simulink model "terrainfollow_debug"  (R2018a)
settings: Solver=VariableStepAuto  StartTime=0.0  StopTime=100  FixedStep=0.00001  RelTol=1e-3
values from neighbouring files (symbols this model uses):
  A = [0 0 0.00013165266625 3.15369085605e-06 -1.52707114267e-20 299.999999993 0 -32.1699999992 -6.02299064272e-14 0 0 0 ... (25 elements, 5x5)]    [redu_ss_terrainfollow.mat]    (also in reducefun_terrainfollow.m = A_lon_ac)
  B = [0  0; 0  0; 0.00154396044469  -0.00453382204302; -9.49308816068e-07  -0.00111635553349; 0  -0.0570163434913]    [redu_ss_terrainfollow.mat]    (also in reducefun_terrainfollow.m = B_lon_ac)
  C = [1 0 0 0 0 0 1 0 0 0 0 0 ... (25 elements, 5x5)]    [redu_ss_terrainfollow.mat]    (also in reducefun_terrainfollow.m = C_lon_ac)
  D = [0  0; 0  0; 0  0; 0  0; 0  0]    [redu_ss_terrainfollow.mat]    (also in reducefun_terrainfollow.m = D_lon_ac)
  ele_lowlim = -25    - de0    [terrainfollow_run.m]    (also in terrainfollow_sim_bigcanyon.m)
  ele_uplim = 25     - de0    [terrainfollow_run.m]    (also in terrainfollow_sim_bigcanyon.m)
  h0 = 1500    [terrainfollow_run.m]    (also in terrainfollow_sim_bigcanyon.m)
  K_f = lqr(A,B,Q_f,R_f)    [terrainfollow_run.m]    (also in terrainfollow_sim_bigcanyon.m)
  th_lowlim = 1000   - th0    [terrainfollow_run.m]    (also in terrainfollow_sim_bigcanyon.m)
  th_uplim = 19000  - th0    [terrainfollow_run.m]    (also in terrainfollow_sim_bigcanyon.m)
  v0 = ft2m*trim_state_lo(7)    [terrainfollow_run.m]    (also in terrainfollow_sim_bigcanyon.m)
libraries: aerolibconvert2 x4
settings Model: Creator=Lukas  LastModifiedBy=Lukas
settings CodeAppCC: StateflowObjectComments=on

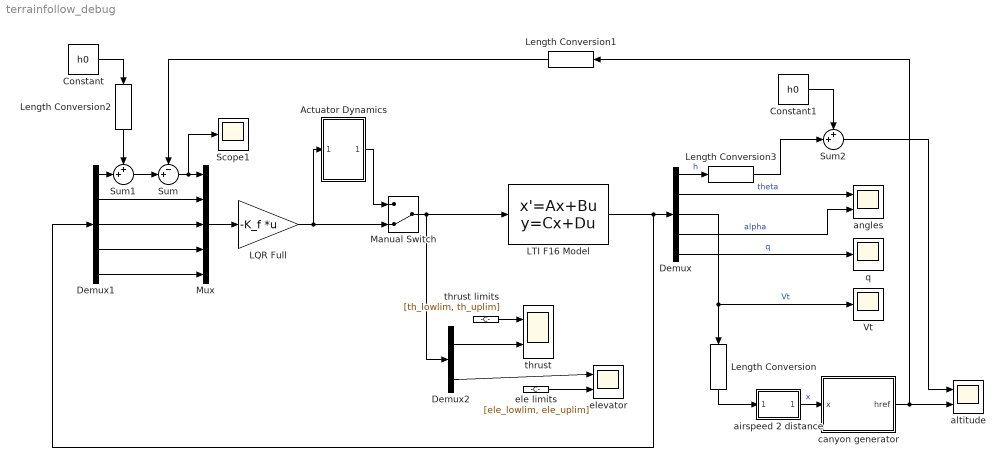
== system terrainfollow_debug ==
  Actuator Dynamics : Subsystem
  Constant : Constant  Value=h0
  Constant1 : Constant  Value=h0
  Demux : Demux  Outputs=5
  Demux1 : Demux  Outputs=5
  Demux2 : Demux  Outputs=2
  LQR Full : Gain  Gain=-K_f  Multiplication=Matrix(K*u)  SaturateOnIntegerOverflow=on  OutDataTypeStr=Inherit: Same as input  ParamDataTypeStr=Inherit: Same as input
  "LTI F16 Model " : StateSpace  A=A  B=B  C=C  D=D  InitialCondition=0
      mask Display: image('f16thumb.jpg');
  Length Conversion : aerolibconvert2/Length Conversion  IU=ft  OU=m
  Length Conversion1 : aerolibconvert2/Length Conversion  IU=m  OU=ft
  Length Conversion2 : aerolibconvert2/Length Conversion  IU=m  OU=ft
  Length Conversion3 : aerolibconvert2/Length Conversion  IU=ft  OU=m
  Manual Switch : ManualSwitch  CurrentSetting=0
  Mux : Mux  Inputs=5
  Scope1 : Scope
  Sum : Sum  Inputs=-+|
  Sum1 : Sum  Inputs=++|
  Sum2 : Sum  Inputs=++|
  Vt : Scope
  airspeed 2 distance : Subsystem
  altitude : Scope  NumInputPorts=2
  angles : Scope  NumInputPorts=2
  canyon generator : Subsystem
      mask Display: image(imread('canyon.jpg'))
  ele limits : Constant  Value=[ele_lowlim, ele_uplim]
  elevator : Scope  NumInputPorts=2
  q : Scope
  thrust : Scope  NumInputPorts=2
  thrust limits : Constant  Value=[th_lowlim, th_uplim]
  wires:
  "LTI F16 Model "/1 -> Demux1/1, Demux/1
  airspeed 2 distance/1(Out1) -> canyon generator/1(x)  "x"
  Demux/2 -> angles/1  "theta"
  Demux/5 -> q/1  "q"
  Demux/1 -> Length Conversion3/1  "h"
  Demux/3 -> Vt/1, Length Conversion/1  "Vt"
  Demux/4 -> angles/2  "alpha"
  Demux1/5 -> Mux/5
  Demux1/3 -> Mux/3
  Demux1/4 -> Mux/4
  Demux1/2 -> Mux/2
  Mux/1 -> LQR Full/1
  Demux1/1 -> Sum1/2
  Sum/1 -> Scope1/1, Mux/1
  canyon generator/1(href) -> Length Conversion1/1, altitude/2
  Sum1/1 -> Sum/2
  Constant/1 -> Length Conversion2/1
  Sum2/1 -> altitude/1
  Constant1/1 -> Sum2/1
  LQR Full/1 -> Manual Switch/2, Actuator Dynamics/1(In1)
  Actuator Dynamics/1(Out1) -> Manual Switch/1
  Manual Switch/1 -> "LTI F16 Model "/1, Demux2/1
  Length Conversion/1 -> airspeed 2 distance/1(In1)
  Length Conversion1/1 -> Sum/1
  Length Conversion2/1 -> Sum1/1
  Length Conversion3/1 -> Sum2/2
  Demux2/1 -> thrust/2
  Demux2/2 -> elevator/1
  thrust limits/1 -> thrust/1
  ele limits/1 -> elevator/2

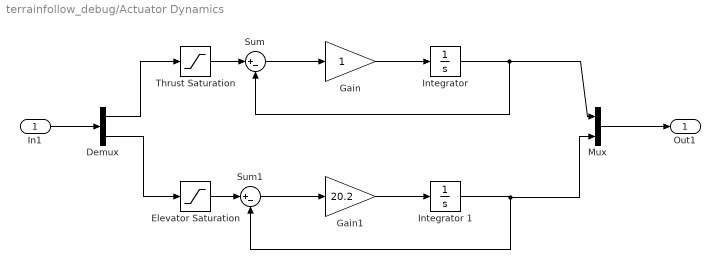
== system terrainfollow_debug/Actuator Dynamics ==
  In1 : Inport
  Demux : Demux  Outputs=2
  Elevator Saturation : Saturate  UpperLimit=ele_uplim  LowerLimit=ele_lowlim
  Gain : Gain  SaturateOnIntegerOverflow=on  OutDataTypeStr=Inherit: Same as input  ParamDataTypeStr=Inherit: Same as input
  Gain1 : Gain  Gain=20.2  SaturateOnIntegerOverflow=on  OutDataTypeStr=Inherit: Same as input  ParamDataTypeStr=Inherit: Same as input
  "Integrator " : Integrator  UpperSaturationLimit=30  LowerSaturationLimit=-30
  Integrator 1 : Integrator  UpperSaturationLimit=25  LowerSaturationLimit=-25
  Mux : Mux  Inputs=2
  Sum : Sum  Inputs=|+-  SaturateOnIntegerOverflow=on  InputSameDT=on  OutDataTypeStr=Inherit: Same as first input
  Sum1 : Sum  Inputs=|+-  SaturateOnIntegerOverflow=on  InputSameDT=on  OutDataTypeStr=Inherit: Same as first input
  Thrust Saturation : Saturate  UpperLimit=th_uplim  LowerLimit=th_lowlim
  Out1 : Outport
  wires:
  Mux/1 -> Out1/1
  In1/1 -> Demux/1
  Sum1/1 -> Gain1/1
  Gain1/1 -> Integrator 1/1
  Integrator 1/1 -> Mux/2, Sum1/2
  Sum/1 -> Gain/1
  "Integrator "/1 -> Mux/1, Sum/2
  Gain/1 -> "Integrator "/1
  Demux/1 -> Thrust Saturation/1
  Demux/2 -> Elevator Saturation/1
  Thrust Saturation/1 -> Sum/1
  Elevator Saturation/1 -> Sum1/1

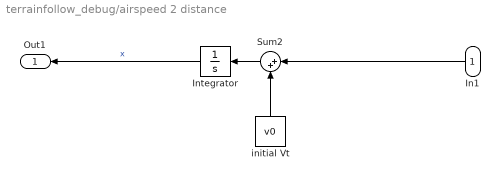
== system terrainfollow_debug/airspeed 2 distance ==
  In1 : Inport
  Integrator : Integrator
  Sum2 : Sum  Inputs=|++
  initial Vt : Constant  Value=v0
  Out1 : Outport
  wires:
  initial Vt/1 -> Sum2/2
  In1/1 -> Sum2/1
  Integrator/1 -> Out1/1  "x"
  Sum2/1 -> Integrator/1

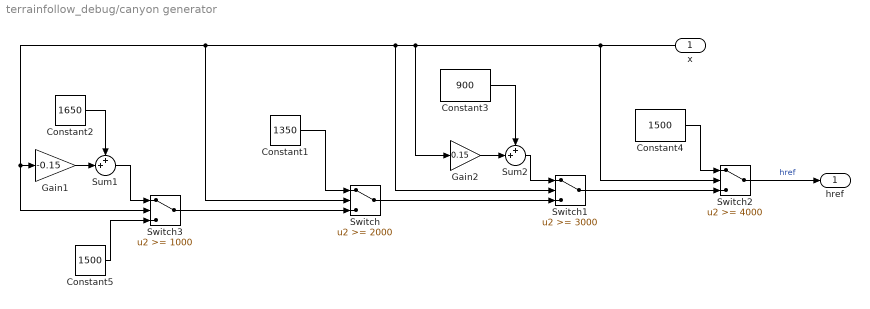
== system terrainfollow_debug/canyon generator ==
  x : Inport
  Constant1 : Constant  Value=1350
  Constant2 : Constant  Value=1650
  Constant3 : Constant  Value=900
  Constant4 : Constant  Value=1500
  Constant5 : Constant  Value=1500
  Gain1 : Gain  Gain=-0.15
  Gain2 : Gain  Gain=0.15
  Sum1 : Sum  Inputs=++|
  Sum2 : Sum  Inputs=++|
  Switch : Switch  Threshold=2000  ZeroCross=off
  Switch1 : Switch  Threshold=3000  ZeroCross=off
  Switch2 : Switch  Threshold=4000  ZeroCross=off
  Switch3 : Switch  Threshold=1000  ZeroCross=off
  href : Outport
  wires:
  Constant1/1 -> Switch/1
  x/1 -> Switch2/2, Gain2/1, Switch1/2, Switch/2, Gain1/1, Switch3/2
  Switch/1 -> Switch1/3
  Gain2/1 -> Sum2/2
  Constant3/1 -> Sum2/1
  Sum2/1 -> Switch1/1
  Switch1/1 -> Switch2/3
  Constant4/1 -> Switch2/1
  Switch2/1 -> href/1  "href"
  Switch3/1 -> Switch/3
  Constant5/1 -> Switch3/3
  Sum1/1 -> Switch3/1
  Gain1/1 -> Sum1/2
  Constant2/1 -> Sum1/1
